simulink model "test_segmented_QA"  (R2018a)
settings: Solver=ode113  StartTime=0.0  StopTime=t(end)  RelTol=1e-6
values from neighbouring files (symbols this model uses):
  K = 1.5e9    (= 1500000000)    [plot_segmented.m]
  r_LU = 12e-3*[1 0.5 0.5 1]    [plot_segmented.m]
libraries: usask_segmented_TLM_lib x1
settings Model: Creator=tkw954  LastModifiedBy=tkw954
settings DataIOCC: ReturnWorkspaceOutputs=on  OutputOption=SpecifiedOutputTimes  OutputTimes=t

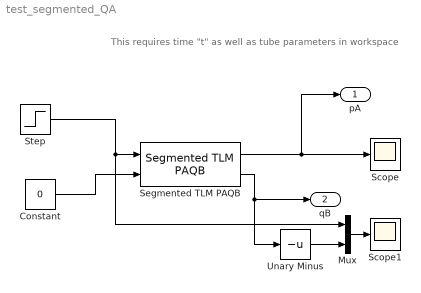
== system test_segmented_QA ==
  note: This requires time "t" as well as tube parameters in workspace
  Constant : Constant  Value=0
  Mux : Mux  Inputs=2
  Scope : Scope
  Scope1 : Scope
  Segmented TLM PAQB : usask_segmented_TLM_lib/Segmented TLM PAQB  x_LU=x_LU  d_LU=2*r_LU  K=K  nu=nu  rho=rho
  Step : Step  Time=0  SampleTime=0
  Unary Minus : UnaryMinus
  pA : Outport
  qB : Outport  Port=2
  wires:
  Constant/1 -> Segmented TLM PAQB/2
  Step/1 -> Segmented TLM PAQB/1, Mux/1
  Segmented TLM PAQB/1 -> pA/1, Scope/1
  Mux/1 -> Scope1/1
  Segmented TLM PAQB/2 -> qB/1, Unary Minus/1
  Unary Minus/1 -> Mux/2
